simulink model "model_SEIRD_UCI_VAC_CEPA"  (R2023a)
settings: Solver=VariableStepAuto  StartTime=0.0  StopTime=1000  RelTol=1e-3
model workspace (MAT data in the model file):
  b = 0.5
  d = 0.02
  g = 0.05
  l = 0.2
  n = 7500000
  ratio_hosp = 0.05
libraries: simulink x1
settings Model: Creator=joans  LastModifiedBy=sergi
settings SolverCC: ZeroCrossControl=DisableAll
settings ModelReferenceCC: EnableRefExpFcnMdlSchedulingChecks=on

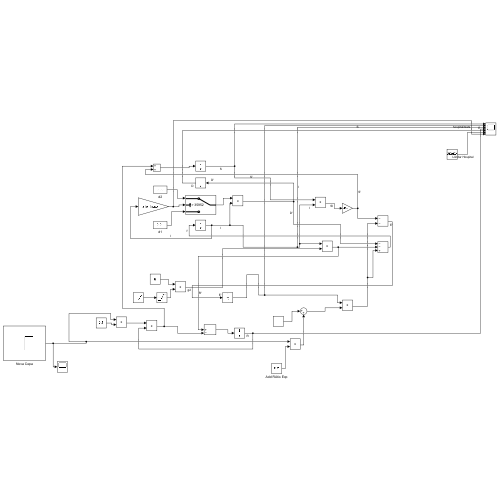
[thumbnail: Simulink's stored preview of the top-level diagram]
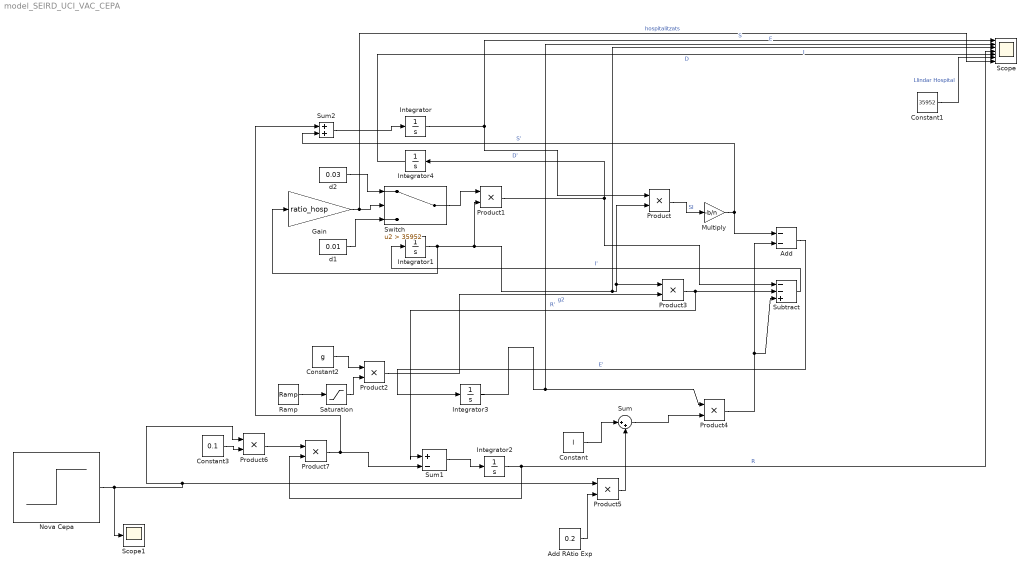
== system model_SEIRD_UCI_VAC_CEPA ==
  Add : Sum  Inputs=--
  Add RAtio Exp : Constant  Value=0.2
  Constant : Constant  Value=l
  Constant1 : Constant  Value=35952
  Constant2 : Constant  Value=g
  Constant3 : Constant  Value=0.1
  Gain : Gain  Gain=ratio_hosp
  Integrator : Integrator  InitialCondition=n
  Integrator1 : Integrator  InitialCondition=10
  Integrator2 : Integrator
  Integrator3 : Integrator
  Integrator4 : Integrator
  Multiply : Gain  Gain=-b/n
  Nova Cepa : Step  Time=100  SampleTime=0
  Product{,1..7} (8 alike) : Product
  Ramp : simulink/Sources/Ramp  slope=0.15  start=50  InitialOutput=1  VectorParams1D=off
  Saturation : Saturate  UpperLimit=5  LowerLimit=0
  Scope : Scope  NumInputPorts=7
  Scope1 : Scope
  Subtract : Sum  Inputs=--+
  Sum : Sum  Inputs=|++
  Sum1 : Sum  Inputs=|+-
  Sum2 : Sum
  Switch : Switch  Criteria=u2 > Threshold  Threshold=35952  SaturateOnIntegerOverflow=off  InputSameDT=off
  d1 : Constant  Value=0.01
  d2 : Constant  Value=0.03
  wires:
  Integrator/1 -> Product/1, Scope/1  "S"
  Integrator1/1 -> Gain/1, Product1/2, Product3/1, Product/2, Scope/3  "I"
  Product/1 -> Multiply/1  "SI"
  Multiply/1 -> Sum2/2, Add/1  "S'"
  Product3/1 -> Sum1/1, Subtract/2  "R'"
  Integrator2/1 -> Product7/2, Scope/4  "R"
  Integrator3/1 -> Scope/2, Product4/1  "E"
  Subtract/1 -> Integrator1/1  "I'"
  Integrator4/1 -> Scope/5  "D"
  Product1/1 -> Subtract/1, Integrator4/1  "D'"
  Product4/1 -> Add/2, Subtract/3
  Add/1 -> Integrator3/1  "E'"
  Switch/1 -> Product1/1
  d2/1 -> Switch/1
  d1/1 -> Switch/3
  Constant1/1 -> Scope/6  "Llindar Hospital"
  Gain/1 -> Scope/7, Switch/2  "hospitalitzats"
  Ramp/1 -> Saturation/1
  Constant2/1 -> Product2/1
  Product2/1 -> Product3/2  "g2"
  Saturation/1 -> Product2/2
  Constant/1 -> Sum/1
  Sum/1 -> Product4/2
  Add RAtio Exp/1 -> Product5/2
  Nova Cepa/1 -> Scope1/1, Product5/1, Product6/1
  Product5/1 -> Sum/2
  Sum1/1 -> Integrator2/1
  Constant3/1 -> Product6/2
  Sum2/1 -> Integrator/1
  Product6/1 -> Product7/1
  Product7/1 -> Sum2/1, Sum1/2
